simulink model "sys_sim_link_act"  (R2021a)
settings: Solver=VariableStepAuto  StartTime=0.0  StopTime=10.0  RelTol=1e-3
settings Model: Creator=Suman  LastModifiedBy=Suman

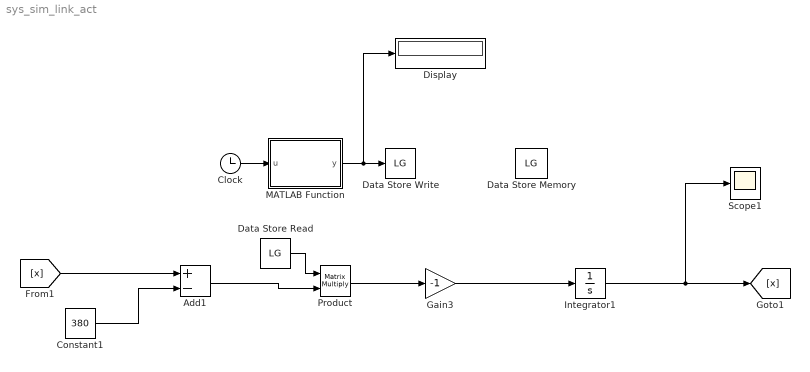
== system sys_sim_link_act ==
  Add1 : Sum  Inputs=+-
  Clock : Clock
  Constant1 : Constant  Value=380
  Data Store Memory : DataStoreMemory  DataStoreName=LG  ReadBeforeWriteMsg=warning  WriteAfterWriteMsg=warning  WriteAfterReadMsg=warning  ShowAdditionalParam=off
  Data Store Read : DataStoreRead  DataStoreName=LG  IndexOptions=Index vector (dialog)  Indices=1  OutputSizes=1
  Data Store Write : DataStoreWrite  DataStoreName=LG  IndexOptions=Index vector (dialog)  Indices=1  OutputSizes=1
  Display : Display
  Gain3 : Gain  Gain=-1
  Integrator1 : Integrator  InitialCondition="[287.1501 ; 145.6127 ; 240.0841 ;  42.5659]"
  MATLAB Function : MATLAB Function  TreatAsAtomicUnit=on
  Product : Product  Multiplication=Matrix(*)
  Scope1 : Scope
  wires:
  Integrator1/1 -> Scope1/1, [x]
  Gain3/1 -> Integrator1/1
  [x] -> Add1/1
  Constant1/1 -> Add1/2
  Add1/1 -> Product/2
  Product/1 -> Gain3/1
  MATLAB Function/1(y) -> Display/1, Data Store Write/1
  Clock/1 -> MATLAB Function/1(u)
  Data Store Read/1 -> Product/1

== matlab function sys_sim_link_act/MATLAB Function ==
  data: u input; y output
function y = fcn(u)
    G=eye(4);
    L=[2 -1 0 -1;-1 2 -1 0;0 -1 2 -1;-1 0 -1 2];
    if u>=10 && u<13
        L(2,4)=500*sin(u);
    else
        L(2,4)=0;
    end
y = L+G;
